simulink model "my_gm_HDLHeaderFull"  (R2024a)
settings: Solver=FixedStepDiscrete  StartTime=0.0  StopTime=stopTime  RelTol=1e-3
values from neighbouring files (symbols this model uses):
  fs = 1    [testHeaderFull.m]
undefined symbols (not defined in the file or in its folder): fPHY, headerBitsPerOFDMSymbol, paramFile
libraries: hdlmdlgenlib x56, simulink x7, dspsrcs4 x5, whdlutilities x5, hdlsllib x3, dspsigops x3, commhdlcrc x1, whdledac x1, HDL_ieee_8021513 x1
settings Model: Creator=cotti  LastModifiedBy=cotti
settings OptimizationCC: BlockReduction=off  ConditionallyExecuteInputs=off  DefaultParameterBehavior=Inlined  InheritOutputTypeSmallerThanSingle=on
settings DebuggingCC: AlgebraicLoopMsg=error  ArtificialAlgebraicLoopMsg=error  InheritedTsInSrcMsg=none  SingleTaskRateTransMsg=error  UnconnectedInputMsg=warning  UnconnectedOutputMsg=warning  UnconnectedLineMsg=warning
settings HardwareCC: ProdBitPerPointer=32  ProdBitPerSizeT=32  ProdBitPerPtrDiffT=32  ProdLargestAtomicFloat=None  ProdIntDivRoundTo=Undefined  ProdEndianess=Unspecified  ProdWordSize=32  ProdHWDeviceType=ASIC/FPGA->ASIC/FPGA  TargetBitPerLong=64  TargetBitPerPointer=64  TargetBitPerSizeT=64  TargetBitPerPtrDiffT=64  TargetLongLongMode=on  TargetIntDivRoundTo=Zero  TargetEndianess=LittleEndian  TargetWordSize=64  TargetHWDeviceType=Custom Processor->MATLAB Host Computer  ProdEqTarget=off

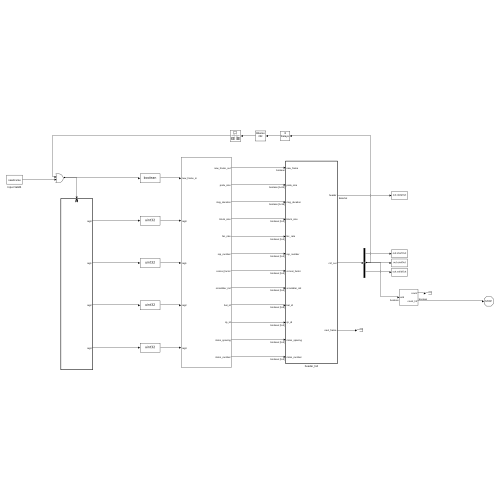
[thumbnail: Simulink's stored preview of the top-level diagram]
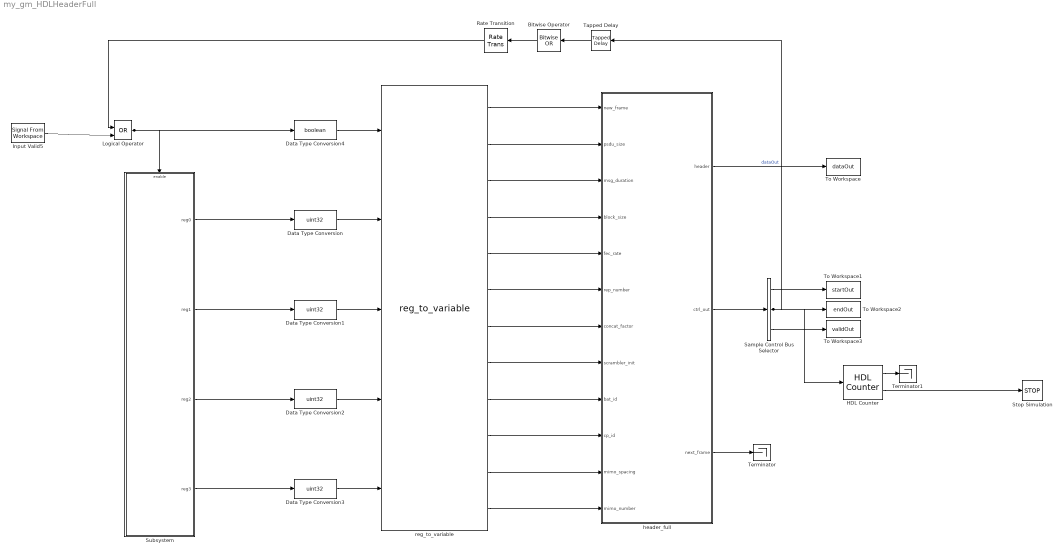
== system my_gm_HDLHeaderFull ==
  Bitwise Operator : simulink/Logic and Bit Operations/Bitwise Operator  logicop=OR  UseBitMask=off  BitMask=bin2dec('11011001')  BitMaskRealWorld=Stored Integer
      settings: LibrarySourceBlock=|
      | hdlsllib/Logic and Bit
      | Operations/Bitwise
      | Operator
  Data Type Conversion{,1..3} (4 alike) : DataTypeConversion  OutDataTypeStr=uint32  SaturateOnIntegerOverflow=off  RndMeth=Floor
  Data Type Conversion4 : DataTypeConversion  OutDataTypeStr=boolean  SaturateOnIntegerOverflow=off  RndMeth=Floor
  HDL Counter : hdlsllib/Sources/HDL Counter  CountType=Count limited  CountInit=0  CountStep=1  CountMax=length(paramFile)  CountFromType=Initial value  CountFrom=0  CountResetPort=off  CountLoadPort=off  CountEnbPort=on  CountDirPort=off  CountHitOutputPort=on  CountDataType=Unsigned  CountWordLen=8  CountFracLen=0  CountSampTime=1
  Input Valid5 : dspsrcs4/Signal From Workspace  X=newFrame  Ts=1/(fPHY/4)  nsamps=1  OutputAfterFinalValue=Setting to zero  ignoreOrWarnInputAndFrameLengths=off  OutputFrames=off
  Logical Operator : Logic  Operator=OR  IconShape=distinctive  AllPortsSameDT=off  OutDataTypeStr=boolean
  Rate Transition : RateTransition  OutPortSampleTimeOpt=Multiple of input port sample time  OutPortSampleTimeMultiple=8
  Sample Control Bus Selector : whdlutilities/Sample Control Bus Selector  OutputSignals=start,end,valid
  Stop Simulation : Stop
  Subsystem : Subsystem
  Tapped Delay : simulink/Discrete/Tapped Delay  vinit=0.0  samptime=-1  NumDelays=8  DelayOrder=Oldest  includeCurrent=off
      settings: LibrarySourceBlock=hdlsllib/Discrete/Tapped Delay
  Terminator : Terminator
  Terminator1 : Terminator
  To Workspace : ToWorkspace  VariableName=dataOut  SampleTime=1/fs
      settings: Save2DSignal=2-D array (concatenate along first dimension)
  To Workspace1 : ToWorkspace  VariableName=startOut  SampleTime=1/fs
      settings: Save2DSignal=2-D array (concatenate along first dimension)
  To Workspace2 : ToWorkspace  VariableName=endOut  SampleTime=1/fs
      settings: Save2DSignal=2-D array (concatenate along first dimension)
  To Workspace3 : ToWorkspace  VariableName=validOut  SampleTime=1/fs
      settings: Save2DSignal=2-D array (concatenate along first dimension)
  header_full : Subsystem  TreatAsAtomicUnit=on
  reg_to_variable : HDL_ieee_8021513/reg_to_variable  SystemSampleTime=-1  VariantActivationTime=update diagram  AllowFlexibleInterface=on  Latency=0  AutoFrameSizeCalculation=off
      settings: SourceProductName=HDL IEEE 8021513
  wires:
  HDL Counter/2 -> Stop Simulation/1
  HDL Counter/1 -> Terminator1/1
  Subsystem/4(reg3) -> Data Type Conversion3/1
  Subsystem/3(reg2) -> Data Type Conversion2/1
  Subsystem/2(reg1) -> Data Type Conversion1/1
  Subsystem/1(reg0) -> Data Type Conversion/1
  Rate Transition/1 -> Logical Operator/1
  Bitwise Operator/1 -> Rate Transition/1
  Tapped Delay/1 -> Bitwise Operator/1
  Input Valid5/1 -> Logical Operator/2
  Logical Operator/1 -> Data Type Conversion4/1, Subsystem/Enable
  header_full/3(next_frame) -> Terminator/1
  Data Type Conversion4/1 -> reg_to_variable/1
  Data Type Conversion3/1 -> reg_to_variable/5
  Data Type Conversion2/1 -> reg_to_variable/4
  Data Type Conversion1/1 -> reg_to_variable/3
  Data Type Conversion/1 -> reg_to_variable/2
  header_full/2(ctrl_out) -> Sample Control Bus Selector/1
  Sample Control Bus Selector/1 -> To Workspace1/1
  Sample Control Bus Selector/3 -> To Workspace3/1
  header_full/1(header) -> To Workspace/1  "dataOut"
  Sample Control Bus Selector/2 -> To Workspace2/1, Tapped Delay/1, HDL Counter/1
  reg_to_variable/1 -> header_full/1(new_frame)
  reg_to_variable/3 -> header_full/3(msg_duration)
  reg_to_variable/4 -> header_full/4(block_size)
  reg_to_variable/5 -> header_full/5(fec_rate)
  reg_to_variable/6 -> header_full/6(rep_number)
  reg_to_variable/7 -> header_full/7(concat_factor)
  reg_to_variable/8 -> header_full/8(scrambler_init)
  reg_to_variable/9 -> header_full/9(bat_id)
  reg_to_variable/10 -> header_full/10(cp_id)
  reg_to_variable/11 -> header_full/11(mimo_spacing)
  reg_to_variable/2 -> header_full/2(psdu_size)
  reg_to_variable/12 -> header_full/12(mimo_number)

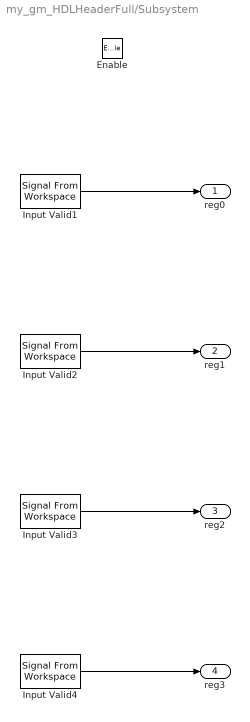
== system my_gm_HDLHeaderFull/Subsystem ==
  Enable : EnablePort
  Input Valid1 : dspsrcs4/Signal From Workspace  X=reg0  Ts=1/(fPHY/4)  nsamps=1  OutputAfterFinalValue=Setting to zero  ignoreOrWarnInputAndFrameLengths=off  OutputFrames=off
  Input Valid2 : dspsrcs4/Signal From Workspace  X=reg1  Ts=1/(fPHY/4)  nsamps=1  OutputAfterFinalValue=Setting to zero  ignoreOrWarnInputAndFrameLengths=off  OutputFrames=off
  Input Valid3 : dspsrcs4/Signal From Workspace  X=reg2  Ts=1/(fPHY/4)  nsamps=1  OutputAfterFinalValue=Setting to zero  ignoreOrWarnInputAndFrameLengths=off  OutputFrames=off
  Input Valid4 : dspsrcs4/Signal From Workspace  X=reg3  Ts=1/(fPHY/4)  nsamps=1  OutputAfterFinalValue=Setting to zero  ignoreOrWarnInputAndFrameLengths=off  OutputFrames=off
  reg0 : Outport
  reg1 : Outport  Port=2
  reg2 : Outport  Port=3
  reg3 : Outport  Port=4
  wires:
  Input Valid1/1 -> reg0/1
  Input Valid4/1 -> reg3/1
  Input Valid2/1 -> reg1/1
  Input Valid3/1 -> reg2/1

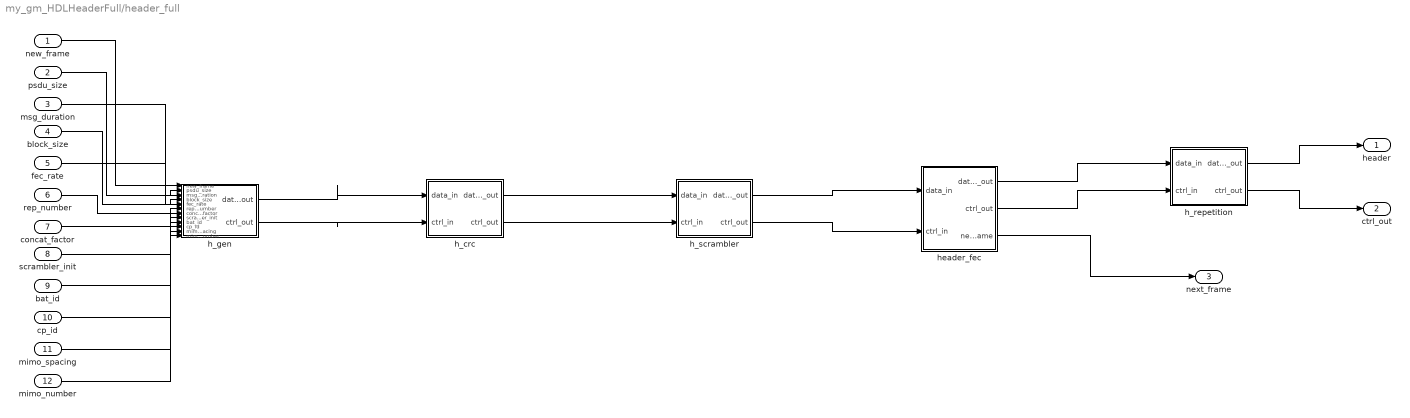
== system my_gm_HDLHeaderFull/header_full ==
  new_frame : Inport  OutDataTypeStr=boolean  SampleTime=8e-08
  psdu_size : Inport  Port=2  OutDataTypeStr=boolean  PortDimensions=[1 24]  SampleTime=8e-08
  msg_duration : Inport  Port=3  OutDataTypeStr=boolean  PortDimensions=[1 16]  SampleTime=8e-08
  block_size : Inport  Port=4  OutDataTypeStr=boolean  PortDimensions=[1 2]  SampleTime=8e-08
  fec_rate : Inport  Port=5  OutDataTypeStr=boolean  PortDimensions=[1 3]  SampleTime=8e-08
  rep_number : Inport  Port=6  OutDataTypeStr=boolean  PortDimensions=[1 3]  SampleTime=8e-08
  concat_factor : Inport  Port=7  OutDataTypeStr=boolean  PortDimensions=[1 3]  SampleTime=8e-08
  scrambler_init : Inport  Port=8  OutDataTypeStr=boolean  PortDimensions=[1 4]  SampleTime=8e-08
  bat_id : Inport  Port=9  OutDataTypeStr=boolean  PortDimensions=[1 5]  SampleTime=8e-08
  cp_id : Inport  Port=10  OutDataTypeStr=boolean  PortDimensions=[1 3]  SampleTime=8e-08
  mimo_spacing : Inport  Port=11  OutDataTypeStr=boolean  PortDimensions=[1 3]  SampleTime=8e-08
  mimo_number : Inport  Port=12  OutDataTypeStr=boolean  PortDimensions=[1 3]  SampleTime=8e-08
  h_crc : Subsystem
  h_gen : Subsystem
  h_repetition : Subsystem
  h_scrambler : Subsystem
  header_fec : Subsystem
  header : Outport  SampleTime=1e-08
  ctrl_out : Outport  Port=2  SampleTime=1e-08
  next_frame : Outport  Port=3  SampleTime=1e-08
  wires:
  new_frame/1 -> h_gen/1(new_frame)
  psdu_size/1 -> h_gen/2(psdu_size)
  msg_duration/1 -> h_gen/3(msg_duration)
  block_size/1 -> h_gen/4(block_size)
  fec_rate/1 -> h_gen/5(fec_rate)
  rep_number/1 -> h_gen/6(rep_number)
  concat_factor/1 -> h_gen/7(concat_factor)
  scrambler_init/1 -> h_gen/8(scrambler_init)
  bat_id/1 -> h_gen/9(bat_id)
  cp_id/1 -> h_gen/10(cp_id)
  mimo_spacing/1 -> h_gen/11(mimo_spacing)
  mimo_number/1 -> h_gen/12(mimo_number)
  h_crc/1(data_out) -> h_scrambler/1(data_in)
  h_crc/2(ctrl_out) -> h_scrambler/2(ctrl_in)
  h_gen/1(data_out) -> h_crc/1(data_in)
  h_gen/2(ctrl_out) -> h_crc/2(ctrl_in)
  h_repetition/1(data_out) -> header/1
  h_repetition/2(ctrl_out) -> ctrl_out/1
  h_scrambler/1(data_out) -> header_fec/1(data_in)
  h_scrambler/2(ctrl_out) -> header_fec/2(ctrl_in)
  header_fec/1(data_out) -> h_repetition/1(data_in)
  header_fec/2(ctrl_out) -> h_repetition/2(ctrl_in)
  header_fec/3(next_frame) -> next_frame/1

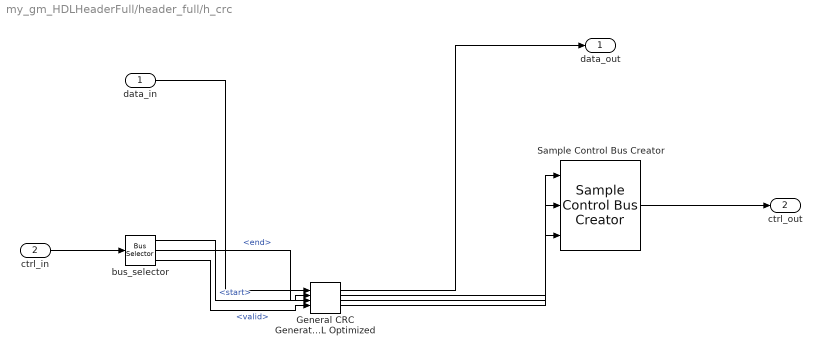
== system my_gm_HDLHeaderFull/header_full/h_crc ==
  data_in : Inport  OutDataTypeStr=boolean  SampleTime=1e-08
  ctrl_in : Inport  Port=2  SampleTime=1e-08
  General CRC Generator HDL Optimized : commhdlcrc/General CRC Generator HDL Optimized  Polynomial=headerCRCPoly  InitialState=1  DirectMethod=on  ReflectInput=off  ReflectCRCChecksum=off  FinalXORValue=0  SimulateUsing=Code generation
  Sample Control Bus Creator : whdlutilities/Sample Control Bus Creator
  bus_selector : BusSelector  OutputSignals=start,end,valid
  data_out : Outport  SampleTime=1e-08
  ctrl_out : Outport  Port=2  SampleTime=1e-08
  wires:
  data_in/1 -> General CRC Generator HDL Optimized/1
  ctrl_in/1 -> bus_selector/1
  General CRC Generator HDL Optimized/1 -> data_out/1
  General CRC Generator HDL Optimized/2 -> Sample Control Bus Creator/1
  General CRC Generator HDL Optimized/3 -> Sample Control Bus Creator/2
  General CRC Generator HDL Optimized/4 -> Sample Control Bus Creator/3
  Sample Control Bus Creator/1 -> ctrl_out/1
  bus_selector/1 -> General CRC Generator HDL Optimized/2  "<start>"
  bus_selector/2 -> General CRC Generator HDL Optimized/3  "<end>"
  bus_selector/3 -> General CRC Generator HDL Optimized/4  "<valid>"

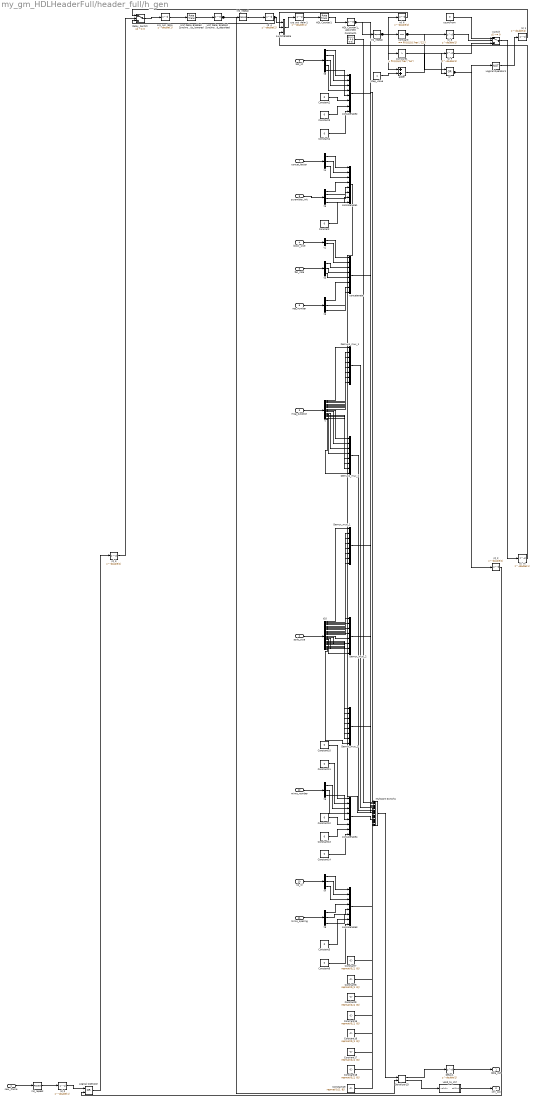
== system my_gm_HDLHeaderFull/header_full/h_gen ==
  new_frame : Inport  OutDataTypeStr=boolean  SampleTime=8e-08
  psdu_size : Inport  Port=2  OutDataTypeStr=boolean  PortDimensions=[1 24]  SampleTime=8e-08
  msg_duration : Inport  Port=3  OutDataTypeStr=boolean  PortDimensions=[1 16]  SampleTime=8e-08
  block_size : Inport  Port=4  OutDataTypeStr=boolean  PortDimensions=[1 2]  SampleTime=8e-08
  fec_rate : Inport  Port=5  OutDataTypeStr=boolean  PortDimensions=[1 3]  SampleTime=8e-08
  rep_number : Inport  Port=6  OutDataTypeStr=boolean  PortDimensions=[1 3]  SampleTime=8e-08
  concat_factor : Inport  Port=7  OutDataTypeStr=boolean  PortDimensions=[1 3]  SampleTime=8e-08
  scrambler_init : Inport  Port=8  OutDataTypeStr=boolean  PortDimensions=[1 4]  SampleTime=8e-08
  bat_id : Inport  Port=9  OutDataTypeStr=boolean  PortDimensions=[1 5]  SampleTime=8e-08
  cp_id : Inport  Port=10  OutDataTypeStr=boolean  PortDimensions=[1 3]  SampleTime=8e-08
  mimo_spacing : Inport  Port=11  OutDataTypeStr=boolean  PortDimensions=[1 3]  SampleTime=8e-08
  mimo_number : Inport  Port=12  OutDataTypeStr=boolean  PortDimensions=[1 3]  SampleTime=8e-08
  Constant{,2..6,10..14} (11 alike) : Constant  Value=0  OutDataTypeStr=boolean  SampleTime=8e-08
  Constant1 : Constant  Value=[0 0 1 1 0 0 0 0]  VectorParams1D=off  OutDataTypeStr=boolean  SampleTime=8e-08
  Constant{7..9,15..19} (8 alike) : Constant  Value="repmat(0,[1  8])"  VectorParams1D=off  OutDataTypeStr=boolean  SampleTime=8e-08
  Delay1 : Delay  DelayLength=double(1)  InitialCondition=0  SampleTime=1e-08
  Delay_Switch : Switch  Criteria=u2 ~= 0  Threshold=double(0)  OutDataTypeStr=boolean  SampleTime=1e-08  SaturateOnIntegerOverflow=off  InputSameDT=off
  Demux1_mux_1 : Mux  Inputs=8
  Demux1_mux_2 : Mux  Inputs=8
  Demux_mux_1 : Mux  Inputs=8
  Demux_mux_2 : Mux  Inputs=8
  Demux_mux_3 : Mux  Inputs=8
  HDL Counter1 : RateTransition  OutPortSampleTimeOpt=Multiple of input port sample time  OutPortSampleTimeMultiple=8
  HDL Counter1_absorbed : Delay  DelayLength=0
  Logical Operator : Logic  Operator=OR  AllPortsSameDT=off  OutDataTypeStr=boolean  SampleTime=1e-08
  Logical Operator1 : Logic  Operator=NOT  Inputs=1  AllPortsSameDT=off  OutDataTypeStr=boolean  SampleTime=1e-08
  Multiport Switch1 : MultiPortSwitch  DataPortOrder=Zero-based contiguous  Inputs=19  DiagnosticForDefault=None  zeroidx=on  SampleTime=8e-08  SaturateOnIntegerOverflow=off  InputSameDT=off
  Serializer1D : hdlsllib/HDL Operations/Serializer1D  Ratio=8  IdleCycles=0  validIn=on  startOut=off  validOut=on  inputDataDimensions=8  inputSampleTime=8e-08  inputSignalType=real
  Unit Delay Enabled Synchronous_lowered : RateTransition  OutPortSampleTimeOpt=Multiple of input port sample time  OutPortSampleTimeMultiple=8
  Unit Delay Enabled Synchronous_lowered_absorbed : Delay  DelayLength=0
  adder : Sum  OutDataTypeStr=fixdt(0, 5, 0)  AccumDataTypeStr=fixdt(0, 5, 0)  SampleTime=1e-08
  compare : simulink/Logic and Bit Operations/Compare To Constant  relop===  const="fi(0,0,5,0,\"hex\",\"12\")"  OutDataTypeStr=boolean
  compare1 : simulink/Logic and Bit Operations/Compare To Constant  relop=>  const="fi(0,0,5,0,\"hex\",\"1e\")"  OutDataTypeStr=boolean
  concatenate{,1..4} (5 alike) : Concatenate  NumInputs=8  Mode=Multidimensional array  ConcatenateDimension=2
  countFrom : Constant  Value=0  VectorParams1D=off  OutDataTypeStr=fixdt(0, 5, 0)  SampleTime=1e-08
  crp_out_delay : Delay  DelayLength=double(1)  InitialCondition=0  SampleTime=1e-08
  crp_out_delay1 : Delay  DelayLength=double(1)  InitialCondition=0  SampleTime=1e-08
  in0_repeat : dspsigops/Repeat  FactorSource=Dialog parameter  N=double(8)  Nmax=16  RateOptions=Allow multirate processing  ic=0  mode=Unused parameter value
  in1_repeat : dspsigops/Repeat  FactorSource=Dialog parameter  N=double(8)  Nmax=16  RateOptions=Allow multirate processing  ic=0  mode=Unused parameter value
  in2_repeat : dspsigops/Repeat  FactorSource=Dialog parameter  N=double(8)  Nmax=16  RateOptions=Allow multirate processing  ic=0  mode=Unused parameter value
  or : Logic  Operator=OR  AllPortsSameDT=off  OutDataTypeStr=boolean  SampleTime=1e-08
  rd_{0,2..3,8..10} (6 alike) : Delay  DelayLength=double(1)  InitialCondition=0  SampleTime=1e-08
  rd_1 : Delay  DelayLength=double(2)  InitialCondition=0  SampleTime=1e-08
  rd_4 : Delay  DelayLength=double(2)  InitialCondition=0  SampleTime=1e-08
  rd_6 : Delay  DelayLength=double(2)  InitialCondition=0  SampleTime=1e-08
  step_value : Constant  VectorParams1D=off  OutDataTypeStr=fixdt(0, 5, 0)  SampleTime=1e-08
  switch : Switch  Criteria=u2 ~= 0  Threshold=double(0)  OutDataTypeStr=fixdt(0, 5, 0)  SampleTime=1e-08  SaturateOnIntegerOverflow=off  InputSameDT=off
  switchEnable : MultiPortSwitch  DataPortOrder=Zero-based contiguous  Inputs=2  DiagnosticForDefault=None  zeroidx=on  OutDataTypeStr=fixdt(0, 5, 0)  SampleTime=1e-08  SaturateOnIntegerOverflow=off  InputSameDT=off
  t : Demux  Outputs=16
  t1 : Demux  Outputs=2
  t10 : Demux  Outputs=24
  t{2..4,7..9} (6 alike) : Demux  Outputs=3
  t5 : Demux
  t6 : Demux  Outputs=5
  valid_to_ctrl : Subsystem
  data_out : Outport  SampleTime=1e-08
  ctrl_out : Outport  Port=2  SampleTime=1e-08
  wires:
  new_frame/1 -> in2_repeat/1
  psdu_size/1 -> t10/1
  msg_duration/1 -> t/1
  block_size/1 -> t1/1
  fec_rate/1 -> t2/1
  rep_number/1 -> t3/1
  concat_factor/1 -> t4/1
  scrambler_init/1 -> t5/1
  bat_id/1 -> t6/1
  cp_id/1 -> t7/1
  mimo_spacing/1 -> t8/1
  mimo_number/1 -> t9/1
  Delay1/1 -> data_out/1
  valid_to_ctrl/1(ctrlOut) -> ctrl_out/1
  Serializer1D/2 -> valid_to_ctrl/1(validIn)
  Serializer1D/1 -> Delay1/1
  Constant1/1 -> Multiport Switch1/2
  Demux1_mux_1/1 -> Multiport Switch1/6
  Demux1_mux_2/1 -> Multiport Switch1/7
  concatenate/1 -> Multiport Switch1/8
  Constant/1 -> concatenate1/8
  concatenate1/1 -> Multiport Switch1/9
  Constant2/1 -> concatenate2/6
  Constant3/1 -> concatenate2/7
  Constant4/1 -> concatenate2/8
  concatenate2/1 -> Multiport Switch1/10
  Constant5/1 -> concatenate3/7
  Constant6/1 -> concatenate3/8
  concatenate3/1 -> Multiport Switch1/11
  Constant7/1 -> Multiport Switch1/12
  Constant8/1 -> Multiport Switch1/13
  Constant9/1 -> Multiport Switch1/14
  Constant10/1 -> concatenate4/1
  Constant11/1 -> concatenate4/2
  Constant12/1 -> concatenate4/6
  Constant13/1 -> concatenate4/7
  Constant14/1 -> concatenate4/8
  concatenate4/1 -> Multiport Switch1/15
  Constant15/1 -> Multiport Switch1/16
  Constant16/1 -> Multiport Switch1/17
  Constant17/1 -> Multiport Switch1/18
  Constant18/1 -> Multiport Switch1/19
  Constant19/1 -> Multiport Switch1/20
  Multiport Switch1/1 -> Serializer1D/1
  Demux_mux_1/1 -> Multiport Switch1/3
  Demux_mux_2/1 -> Multiport Switch1/4
  Demux_mux_3/1 -> Multiport Switch1/5
  t/1 -> Demux1_mux_1/1
  t/2 -> Demux1_mux_1/2
  t/3 -> Demux1_mux_1/3
  t/4 -> Demux1_mux_1/4
  t/5 -> Demux1_mux_1/5
  t/6 -> Demux1_mux_1/6
  t/7 -> Demux1_mux_1/7
  t/8 -> Demux1_mux_1/8
  t/9 -> Demux1_mux_2/1
  t/10 -> Demux1_mux_2/2
  t/11 -> Demux1_mux_2/3
  t/12 -> Demux1_mux_2/4
  t/13 -> Demux1_mux_2/5
  t/14 -> Demux1_mux_2/6
  t/15 -> Demux1_mux_2/7
  t/16 -> Demux1_mux_2/8
  t1/1 -> concatenate/1
  t1/2 -> concatenate/2
  t2/1 -> concatenate/3
  t2/2 -> concatenate/4
  t2/3 -> concatenate/5
  t3/1 -> concatenate/6
  t3/2 -> concatenate/7
  t3/3 -> concatenate/8
  t4/1 -> concatenate1/1
  t4/2 -> concatenate1/2
  t4/3 -> concatenate1/3
  t5/1 -> concatenate1/4
  t5/2 -> concatenate1/5
  t5/3 -> concatenate1/6
  t5/4 -> concatenate1/7
  t6/1 -> concatenate2/1
  t6/2 -> concatenate2/2
  t6/3 -> concatenate2/3
  t6/4 -> concatenate2/4
  t6/5 -> concatenate2/5
  t7/1 -> concatenate3/1
  t7/2 -> concatenate3/2
  t7/3 -> concatenate3/3
  t8/1 -> concatenate3/4
  t8/2 -> concatenate3/5
  t8/3 -> concatenate3/6
  t9/1 -> concatenate4/3
  t9/2 -> concatenate4/4
  t9/3 -> concatenate4/5
  t10/1 -> Demux_mux_1/1
  t10/2 -> Demux_mux_1/2
  t10/3 -> Demux_mux_1/3
  t10/4 -> Demux_mux_1/4
  t10/5 -> Demux_mux_1/5
  t10/6 -> Demux_mux_1/6
  t10/7 -> Demux_mux_1/7
  t10/8 -> Demux_mux_1/8
  t10/9 -> Demux_mux_2/1
  t10/10 -> Demux_mux_2/2
  t10/11 -> Demux_mux_2/3
  t10/12 -> Demux_mux_2/4
  t10/13 -> Demux_mux_2/5
  t10/14 -> Demux_mux_2/6
  t10/15 -> Demux_mux_2/7
  t10/16 -> Demux_mux_2/8
  t10/17 -> Demux_mux_3/1
  t10/18 -> Demux_mux_3/2
  t10/19 -> Demux_mux_3/3
  t10/20 -> Demux_mux_3/4
  t10/21 -> Demux_mux_3/5
  t10/22 -> Demux_mux_3/6
  t10/23 -> Demux_mux_3/7
  t10/24 -> Demux_mux_3/8
  Unit Delay Enabled Synchronous_lowered_absorbed/1 -> Serializer1D/2, in0_repeat/1
  in2_repeat/1 -> rd_0/1
  HDL Counter1/1 -> HDL Counter1_absorbed/1
  HDL Counter1_absorbed/1 -> Multiport Switch1/1, in1_repeat/1
  in1_repeat/1 -> rd_6/1, adder/1, compare/1, compare1/1
  in0_repeat/1 -> rd_4/1
  crp_out_delay/1 -> Unit Delay Enabled Synchronous_lowered/1
  crp_out_delay1/1 -> HDL Counter1/1
  Unit Delay Enabled Synchronous_lowered/1 -> Unit Delay Enabled Synchronous_lowered_absorbed/1
  switchEnable/1 -> crp_out_delay1/1
  countFrom/1 -> switch/1
  step_value/1 -> adder/2
  adder/1 -> rd_9/1
  switch/1 -> rd_10/1
  compare/1 -> rd_8/1, or/1
  compare1/1 -> or/2
  or/1 -> rd_2/1, Logical Operator1/1
  Logical Operator1/1 -> rd_1/1
  Delay_Switch/1 -> crp_out_delay/1
  Logical Operator/1 -> rd_3/1
  rd_6/1 -> switchEnable/2
  rd_1/1 -> Delay_Switch/1
  rd_0/1 -> Logical Operator/1
  rd_2/1 -> Logical Operator/2
  rd_3/1 -> Delay_Switch/2
  rd_9/1 -> switch/3
  rd_10/1 -> switchEnable/3
  rd_8/1 -> switch/2
  rd_4/1 -> Delay_Switch/3, switchEnable/1

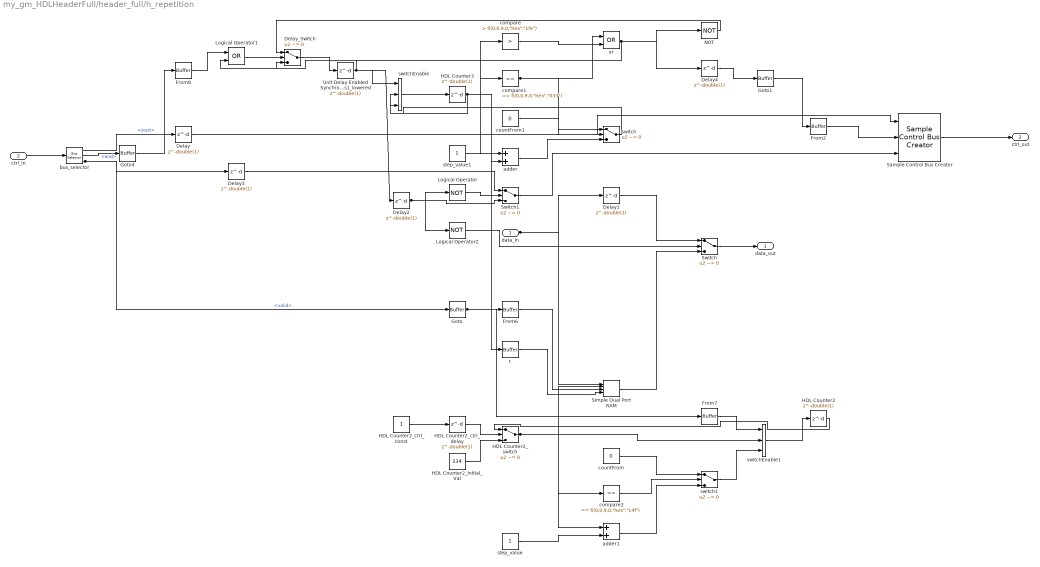
== system my_gm_HDLHeaderFull/header_full/h_repetition ==
  data_in : Inport  OutDataTypeStr=boolean  SampleTime=1e-08
  ctrl_in : Inport  Port=2  SampleTime=1e-08
  Delay{,1..4} (5 alike) : Delay  DelayLength=double(1)  InitialCondition=0  SampleTime=1e-08
  Delay_Switch : Switch  Criteria=u2 ~= 0  Threshold=double(0)  OutDataTypeStr=boolean  SampleTime=1e-08  SaturateOnIntegerOverflow=off  InputSameDT=off
  From{2,6..8} (4 alike) : hdlmdlgenlib/Buffer
  Goto : hdlmdlgenlib/Buffer
  Goto1 : hdlmdlgenlib/Buffer
  Goto4 : hdlmdlgenlib/Buffer
  HDL Counter2 : Delay  DelayLength=double(1)  InitialCondition=0  SampleTime=1e-08
  HDL Counter2_Initial_Val : Constant  Value=334  OutDataTypeStr=fixdt(0, 9, 0)  SampleTime=1e-08
  HDL Counter2_ctrl_const : Constant  OutDataTypeStr=boolean  SampleTime=1e-08
  HDL Counter2_ctrl_delay : Delay  DelayLength=double(1)  InitialCondition=0  SampleTime=1e-08
  HDL Counter2_switch : Switch  Criteria=u2 ~= 0  Threshold=double(0)  OutDataTypeStr=fixdt(0, 9, 0)  SampleTime=1e-08  SaturateOnIntegerOverflow=off  InputSameDT=off
  HDL Counter3 : Delay  DelayLength=double(1)  InitialCondition=0  SampleTime=1e-08
  Logical Operator : Logic  Operator=NOT  Inputs=1  AllPortsSameDT=off  OutDataTypeStr=boolean  SampleTime=1e-08
  Logical Operator1 : Logic  Operator=OR  AllPortsSameDT=off  OutDataTypeStr=boolean  SampleTime=1e-08
  Logical Operator2 : Logic  Operator=NOT  Inputs=1  AllPortsSameDT=off  OutDataTypeStr=boolean  SampleTime=1e-08
  NOT : Logic  Operator=NOT  Inputs=1  AllPortsSameDT=off  OutDataTypeStr=boolean  SampleTime=1e-08
  Sample Control Bus Creator : whdlutilities/Sample Control Bus Creator
  Simple Dual Port RAM : hdlsllib/HDL RAMs/Simple Dual Port RAM  ram_size=nextpow2(headerBitsPerOFDMSymbol)
  Switch : Switch  Criteria=u2 ~= 0  Threshold=double(0)  OutDataTypeStr=boolean  SampleTime=1e-08  SaturateOnIntegerOverflow=off  InputSameDT=off
  Switch1 : Switch  Criteria=u2 ~= 0  Threshold=double(0)  OutDataTypeStr=boolean  SampleTime=1e-08  SaturateOnIntegerOverflow=off  InputSameDT=off
  Unit Delay Enabled Synchronous1_lowered : Delay  DelayLength=double(1)  InitialCondition=0  SampleTime=1e-08
  adder : Sum  OutDataTypeStr=fixdt(0, 9, 0)  AccumDataTypeStr=fixdt(0, 9, 0)  SampleTime=1e-08
  adder1 : Sum  OutDataTypeStr=fixdt(0, 9, 0)  AccumDataTypeStr=fixdt(0, 9, 0)  SampleTime=1e-08
  bus_selector : BusSelector  OutputSignals=start,end,valid
  compare : simulink/Logic and Bit Operations/Compare To Constant  relop=>  const="fi(0,0,9,0,\"hex\",\"1fe\")"  OutDataTypeStr=boolean
  compare1 : simulink/Logic and Bit Operations/Compare To Constant  relop===  const="fi(0,0,9,0,\"hex\",\"033\")"  OutDataTypeStr=boolean
  compare2 : simulink/Logic and Bit Operations/Compare To Constant  relop===  const="fi(0,0,9,0,\"hex\",\"14f\")"  OutDataTypeStr=boolean
  countFrom : Constant  Value=0  VectorParams1D=off  OutDataTypeStr=fixdt(0, 9, 0)  SampleTime=1e-08
  countFrom1 : Constant  Value=0  VectorParams1D=off  OutDataTypeStr=fixdt(0, 9, 0)  SampleTime=1e-08
  or : Logic  Operator=OR  AllPortsSameDT=off  OutDataTypeStr=boolean  SampleTime=1e-08
  step_value : Constant  VectorParams1D=off  OutDataTypeStr=fixdt(0, 9, 0)  SampleTime=1e-08
  step_value1 : Constant  VectorParams1D=off  OutDataTypeStr=fixdt(0, 9, 0)  SampleTime=1e-08
  switch : Switch  Criteria=u2 ~= 0  Threshold=double(0)  OutDataTypeStr=fixdt(0, 9, 0)  SampleTime=1e-08  SaturateOnIntegerOverflow=off  InputSameDT=off
  switch1 : Switch  Criteria=u2 ~= 0  Threshold=double(0)  OutDataTypeStr=fixdt(0, 9, 0)  SampleTime=1e-08  SaturateOnIntegerOverflow=off  InputSameDT=off
  switchEnable : MultiPortSwitch  DataPortOrder=Zero-based contiguous  Inputs=2  DiagnosticForDefault=None  zeroidx=on  OutDataTypeStr=fixdt(0, 9, 0)  SampleTime=1e-08  SaturateOnIntegerOverflow=off  InputSameDT=off
  switchEnable1 : MultiPortSwitch  DataPortOrder=Zero-based contiguous  Inputs=2  DiagnosticForDefault=None  zeroidx=on  OutDataTypeStr=fixdt(0, 9, 0)  SampleTime=1e-08  SaturateOnIntegerOverflow=off  InputSameDT=off
  t : hdlmdlgenlib/Buffer
  data_out : Outport  SampleTime=1e-08
  ctrl_out : Outport  Port=2  SampleTime=1e-08
  wires:
  data_in/1 -> Delay1/1, Simple Dual Port RAM/1
  ctrl_in/1 -> bus_selector/1
  bus_selector/1 -> Delay/1  "<start>"
  bus_selector/2 -> Goto4/1  "<end>"
  bus_selector/3 -> Goto/1, Delay3/1  "<valid>"
  Delay/1 -> Sample Control Bus Creator/1
  Delay1/1 -> Switch/1
  Delay2/1 -> Switch1/3, Logical Operator2/1, Logical Operator/1
  Delay3/1 -> Switch1/1
  Delay4/1 -> Goto1/1
  From2/1 -> Sample Control Bus Creator/2
  From6/1 -> Simple Dual Port RAM/3
  From7/1 -> switchEnable1/1
  t/1 -> Simple Dual Port RAM/4
  Logical Operator/1 -> Switch1/2
  Logical Operator2/1 -> Switch/2
  Sample Control Bus Creator/1 -> ctrl_out/1
  Simple Dual Port RAM/1 -> Switch/3
  Switch/1 -> data_out/1
  Switch1/1 -> Sample Control Bus Creator/3
  Unit Delay Enabled Synchronous1_lowered/1 -> Delay2/1, switchEnable/1, Delay_Switch/3
  Goto1/1 -> From2/1
  Goto/1 -> From7/1, From6/1
  Goto4/1 -> From8/1
  HDL Counter2_switch/1 -> adder1/1, compare2/1, switchEnable1/2, Simple Dual Port RAM/2
  HDL Counter3/1 -> t/1, adder/1, compare1/1, compare/1, switchEnable/2
  or/1 -> Delay4/1, Logical Operator1/2, NOT/1
  HDL Counter2_ctrl_const/1 -> HDL Counter2_ctrl_delay/1
  step_value1/1 -> adder/2
  countFrom1/1 -> switch/1
  From8/1 -> Logical Operator1/1
  Delay_Switch/1 -> Unit Delay Enabled Synchronous1_lowered/1
  switchEnable/1 -> HDL Counter3/1
  adder/1 -> switch/3
  switch/1 -> switchEnable/3
  Logical Operator1/1 -> Delay_Switch/2
  compare/1 -> or/2
  compare1/1 -> or/1, switch/2
  NOT/1 -> Delay_Switch/1
  HDL Counter2/1 -> HDL Counter2_switch/1
  step_value/1 -> adder1/2
  countFrom/1 -> switch1/1
  HDL Counter2_ctrl_delay/1 -> HDL Counter2_switch/2
  HDL Counter2_Initial_Val/1 -> HDL Counter2_switch/3
  switchEnable1/1 -> HDL Counter2/1
  adder1/1 -> switch1/3
  compare2/1 -> switch1/2
  switch1/1 -> switchEnable1/3

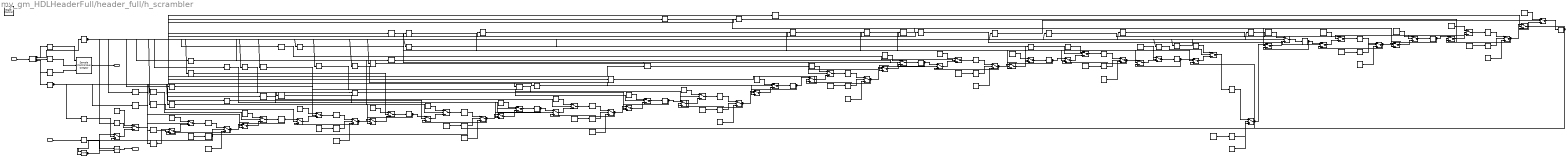
== system my_gm_HDLHeaderFull/header_full/h_scrambler ==
  data_in : Inport  OutDataTypeStr=boolean  SampleTime=1e-08
  ctrl_in : Inport  Port=2  SampleTime=1e-08
  C10_lowered : Delay  DelayLength=double(1)  InitialCondition=0  SampleTime=1e-08
  C10_lowered_Initial_Val : Constant  Value=double(1)  OutDataTypeStr=boolean  SampleTime=1e-08
  C10_lowered_ctrl_const : Constant  OutDataTypeStr=boolean  SampleTime=1e-08
  C10_lowered_ctrl_delay : Delay  DelayLength=double(1)  InitialCondition=0  SampleTime=1e-08
  C10_lowered_switch : Switch  Criteria=u2 ~= 0  Threshold=double(0)  OutDataTypeStr=boolean  SampleTime=1e-08  SaturateOnIntegerOverflow=off  InputSameDT=off
  C11_lowered : Delay  DelayLength=double(1)  InitialCondition=0  SampleTime=1e-08
  C12_lowered : Delay  DelayLength=double(1)  InitialCondition=0  SampleTime=1e-08
  C12_lowered_Initial_Val : Constant  Value=double(1)  OutDataTypeStr=boolean  SampleTime=1e-08
  C12_lowered_ctrl_const : Constant  OutDataTypeStr=boolean  SampleTime=1e-08
  C12_lowered_ctrl_delay : Delay  DelayLength=double(1)  InitialCondition=0  SampleTime=1e-08
  C12_lowered_switch : Switch  Criteria=u2 ~= 0  Threshold=double(0)  OutDataTypeStr=boolean  SampleTime=1e-08  SaturateOnIntegerOverflow=off  InputSameDT=off
  C13_lowered : Delay  DelayLength=double(1)  InitialCondition=0  SampleTime=1e-08
  C14_lowered : Delay  DelayLength=double(1)  InitialCondition=0  SampleTime=1e-08
  C14_lowered_Initial_Val : Constant  Value=double(1)  OutDataTypeStr=boolean  SampleTime=1e-08
  C14_lowered_ctrl_const : Constant  OutDataTypeStr=boolean  SampleTime=1e-08
  C14_lowered_ctrl_delay : Delay  DelayLength=double(1)  InitialCondition=0  SampleTime=1e-08
  C14_lowered_switch : Switch  Criteria=u2 ~= 0  Threshold=double(0)  OutDataTypeStr=boolean  SampleTime=1e-08  SaturateOnIntegerOverflow=off  InputSameDT=off
  C15_lowered : Delay  DelayLength=double(1)  InitialCondition=0  SampleTime=1e-08
  C16_lowered : Delay  DelayLength=double(1)  InitialCondition=0  SampleTime=1e-08
  C16_lowered_Initial_Val : Constant  Value=double(1)  OutDataTypeStr=boolean  SampleTime=1e-08
  C16_lowered_ctrl_const : Constant  OutDataTypeStr=boolean  SampleTime=1e-08
  C16_lowered_ctrl_delay : Delay  DelayLength=double(1)  InitialCondition=0  SampleTime=1e-08
  C16_lowered_switch : Switch  Criteria=u2 ~= 0  Threshold=double(0)  OutDataTypeStr=boolean  SampleTime=1e-08  SaturateOnIntegerOverflow=off  InputSameDT=off
  C17_lowered : Delay  DelayLength=double(1)  InitialCondition=0  SampleTime=1e-08
  C18_lowered : Delay  DelayLength=double(1)  InitialCondition=0  SampleTime=1e-08
  C18_lowered_Initial_Val : Constant  Value=double(1)  OutDataTypeStr=boolean  SampleTime=1e-08
  C18_lowered_ctrl_const : Constant  OutDataTypeStr=boolean  SampleTime=1e-08
  C18_lowered_ctrl_delay : Delay  DelayLength=double(1)  InitialCondition=0  SampleTime=1e-08
  C18_lowered_switch : Switch  Criteria=u2 ~= 0  Threshold=double(0)  OutDataTypeStr=boolean  SampleTime=1e-08  SaturateOnIntegerOverflow=off  InputSameDT=off
  C19_lowered : Delay  DelayLength=double(1)  InitialCondition=0  SampleTime=1e-08
  C1_lowered : Delay  DelayLength=double(1)  InitialCondition=0  SampleTime=1e-08
  C20_lowered : Delay  DelayLength=double(1)  InitialCondition=0  SampleTime=1e-08
  C20_lowered_Initial_Val : Constant  Value=double(1)  OutDataTypeStr=boolean  SampleTime=1e-08
  C20_lowered_ctrl_const : Constant  OutDataTypeStr=boolean  SampleTime=1e-08
  C20_lowered_ctrl_delay : Delay  DelayLength=double(1)  InitialCondition=0  SampleTime=1e-08
  C20_lowered_switch : Switch  Criteria=u2 ~= 0  Threshold=double(0)  OutDataTypeStr=boolean  SampleTime=1e-08  SaturateOnIntegerOverflow=off  InputSameDT=off
  C21_lowered : Delay  DelayLength=double(1)  InitialCondition=0  SampleTime=1e-08
  C22_lowered : Delay  DelayLength=double(1)  InitialCondition=0  SampleTime=1e-08
  C22_lowered_Initial_Val : Constant  Value=double(1)  OutDataTypeStr=boolean  SampleTime=1e-08
  C22_lowered_ctrl_const : Constant  OutDataTypeStr=boolean  SampleTime=1e-08
  C22_lowered_ctrl_delay : Delay  DelayLength=double(1)  InitialCondition=0  SampleTime=1e-08
  C22_lowered_switch : Switch  Criteria=u2 ~= 0  Threshold=double(0)  OutDataTypeStr=boolean  SampleTime=1e-08  SaturateOnIntegerOverflow=off  InputSameDT=off
  C23_lowered : Delay  DelayLength=double(1)  InitialCondition=0  SampleTime=1e-08
  C2_lowered : Delay  DelayLength=double(1)  InitialCondition=0  SampleTime=1e-08
  C2_lowered_Initial_Val : Constant  Value=double(1)  OutDataTypeStr=boolean  SampleTime=1e-08
  C2_lowered_ctrl_const : Constant  OutDataTypeStr=boolean  SampleTime=1e-08
  C2_lowered_ctrl_delay : Delay  DelayLength=double(1)  InitialCondition=0  SampleTime=1e-08
  C2_lowered_switch : Switch  Criteria=u2 ~= 0  Threshold=double(0)  OutDataTypeStr=boolean  SampleTime=1e-08  SaturateOnIntegerOverflow=off  InputSameDT=off
  C3_lowered : Delay  DelayLength=double(1)  InitialCondition=0  SampleTime=1e-08
  C4_lowered : Delay  DelayLength=double(1)  InitialCondition=0  SampleTime=1e-08
  C4_lowered_Initial_Val : Constant  Value=double(1)  OutDataTypeStr=boolean  SampleTime=1e-08
  C4_lowered_ctrl_const : Constant  OutDataTypeStr=boolean  SampleTime=1e-08
  C4_lowered_ctrl_delay : Delay  DelayLength=double(1)  InitialCondition=0  SampleTime=1e-08
  C4_lowered_switch : Switch  Criteria=u2 ~= 0  Threshold=double(0)  OutDataTypeStr=boolean  SampleTime=1e-08  SaturateOnIntegerOverflow=off  InputSameDT=off
  C5_lowered : Delay  DelayLength=double(1)  InitialCondition=0  SampleTime=1e-08
  C6_lowered : Delay  DelayLength=double(1)  InitialCondition=0  SampleTime=1e-08
  C6_lowered_Initial_Val : Constant  Value=double(1)  OutDataTypeStr=boolean  SampleTime=1e-08
  C6_lowered_ctrl_const : Constant  OutDataTypeStr=boolean  SampleTime=1e-08
  C6_lowered_ctrl_delay : Delay  DelayLength=double(1)  InitialCondition=0  SampleTime=1e-08
  C6_lowered_switch : Switch  Criteria=u2 ~= 0  Threshold=double(0)  OutDataTypeStr=boolean  SampleTime=1e-08  SaturateOnIntegerOverflow=off  InputSameDT=off
  C7_lowered : Delay  DelayLength=double(1)  InitialCondition=0  SampleTime=1e-08
  C8_lowered : Delay  DelayLength=double(1)  InitialCondition=0  SampleTime=1e-08
  C8_lowered_Initial_Val : Constant  Value=double(1)  OutDataTypeStr=boolean  SampleTime=1e-08
  C8_lowered_ctrl_const : Constant  OutDataTypeStr=boolean  SampleTime=1e-08
  C8_lowered_ctrl_delay : Delay  DelayLength=double(1)  InitialCondition=0  SampleTime=1e-08
  C8_lowered_switch : Switch  Criteria=u2 ~= 0  Threshold=double(0)  OutDataTypeStr=boolean  SampleTime=1e-08  SaturateOnIntegerOverflow=off  InputSameDT=off
  C9_lowered : Delay  DelayLength=double(1)  InitialCondition=0  SampleTime=1e-08
  Delay{1,3..5} (4 alike) : Delay  DelayLength=double(1)  InitialCondition=0  SampleTime=1e-08
  From{1..46} (46 alike) : hdlmdlgenlib/Buffer
  Goto2 : hdlmdlgenlib/Buffer
  Goto3 : hdlmdlgenlib/Buffer
  Initial_Val{,2,4,6,8,10,13,15..16,18,20,22} (12 alike) : Constant  Value=double(0)  OutDataTypeStr=boolean  SampleTime=1e-08
  Initial_Val{1,3,5,7,9,11..12,14,17,19,21} (11 alike) : Constant  Value=double(1)  OutDataTypeStr=boolean  SampleTime=1e-08
  Logical Operator : Logic  Operator=XOR  AllPortsSameDT=off  OutDataTypeStr=boolean  SampleTime=1e-08
  Logical Operator1 : Logic  Operator=XOR  AllPortsSameDT=off  OutDataTypeStr=boolean  SampleTime=1e-08
  Sample Control Bus Creator : whdlutilities/Sample Control Bus Creator
  StateControl : StateControl  StateControl=Synchronous
  bus_selector : BusSelector  OutputSignals=start,end,valid
  enb_in{,1..22} (23 alike) : Switch  Criteria=u2 ~= 0  Threshold=double(0)  OutDataTypeStr=boolean  SampleTime=1e-08  SaturateOnIntegerOverflow=off  InputSameDT=off
  reset_in{,1..22} (23 alike) : Switch  Criteria=u2 ~= 0  Threshold=double(0)  OutDataTypeStr=boolean  SampleTime=1e-08  SaturateOnIntegerOverflow=off  InputSameDT=off
  data_out : Outport  SampleTime=1e-08
  ctrl_out : Outport  Port=2  SampleTime=1e-08
  wires:
  data_in/1 -> Delay1/1
  ctrl_in/1 -> bus_selector/1
  bus_selector/1 -> Goto3/1, Delay3/1  "<start>"
  bus_selector/2 -> Delay4/1  "<end>"
  bus_selector/3 -> Goto2/1, Delay5/1  "<valid>"
  Delay1/1 -> Logical Operator/1
  Delay3/1 -> Sample Control Bus Creator/1
  Delay4/1 -> Sample Control Bus Creator/2
  Delay5/1 -> Sample Control Bus Creator/3
  Logical Operator/1 -> data_out/1
  Logical Operator1/1 -> Logical Operator/2, enb_in/1
  Sample Control Bus Creator/1 -> ctrl_out/1
  Goto2/1 -> From8/1, From7/1, From5/1, From44/1, From42/1, From40/1, From38/1, From36/1, From34/1, From32/1, From30/1, From3/1, From28/1, From26/1, From24/1, From22/1, From20/1, From18/1, From16/1, From14/1, From12/1, From10/1, From1/1
  Goto3/1 -> From9/1, From6/1, From46/1, From45/1, From43/1, From41/1, From4/1, From39/1, From37/1, From35/1, From33/1, From31/1, From29/1, From27/1, From25/1, From23/1, From21/1, From2/1, From19/1, From17/1, From15/1, From13/1, From11/1
  C10_lowered_ctrl_const/1 -> C10_lowered_ctrl_delay/1
  C12_lowered_ctrl_const/1 -> C12_lowered_ctrl_delay/1
  C14_lowered_ctrl_const/1 -> C14_lowered_ctrl_delay/1
  C16_lowered_ctrl_const/1 -> C16_lowered_ctrl_delay/1
  C18_lowered_ctrl_const/1 -> C18_lowered_ctrl_delay/1
  C2_lowered_ctrl_const/1 -> C2_lowered_ctrl_delay/1
  C20_lowered_ctrl_const/1 -> C20_lowered_ctrl_delay/1
  C22_lowered_ctrl_const/1 -> C22_lowered_ctrl_delay/1
  C4_lowered_ctrl_const/1 -> C4_lowered_ctrl_delay/1
  C6_lowered_ctrl_const/1 -> C6_lowered_ctrl_delay/1
  C8_lowered_ctrl_const/1 -> C8_lowered_ctrl_delay/1
  C1_lowered/1 -> enb_in3/1, enb_in/3
  C19_lowered/1 -> enb_in5/1, enb_in2/3
  C3_lowered/1 -> enb_in7/1, enb_in4/3
  C21_lowered/1 -> enb_in9/1, enb_in6/3
  C5_lowered/1 -> enb_in11/1, enb_in8/3
  C23_lowered/1 -> enb_in10/3, Logical Operator1/1
  C7_lowered/1 -> enb_in13/1, enb_in12/3
  C9_lowered/1 -> enb_in15/1, enb_in14/3
  C11_lowered/1 -> enb_in17/1, enb_in16/3
  C13_lowered/1 -> enb_in19/1, enb_in18/3
  C15_lowered/1 -> enb_in21/1, enb_in20/3
  C17_lowered/1 -> enb_in22/3, enb_in1/1
  C18_lowered/1 -> C18_lowered_switch/1
  From7/1 -> enb_in/2
  Initial_Val/1 -> reset_in/1
  From46/1 -> reset_in/2
  From40/1 -> enb_in1/2
  Initial_Val9/1 -> reset_in1/1
  From41/1 -> reset_in1/2
  C18_lowered_ctrl_delay/1 -> C18_lowered_switch/2
  C18_lowered_Initial_Val/1 -> C18_lowered_switch/3
  From42/1 -> enb_in2/2
  Initial_Val10/1 -> reset_in2/1
  From43/1 -> reset_in2/2
  C2_lowered/1 -> C2_lowered_switch/1
  From1/1 -> enb_in3/2
  Initial_Val11/1 -> reset_in3/1
  From2/1 -> reset_in3/2
  C2_lowered_ctrl_delay/1 -> C2_lowered_switch/2
  C2_lowered_Initial_Val/1 -> C2_lowered_switch/3
  From3/1 -> enb_in4/2
  Initial_Val16/1 -> reset_in4/1
  From4/1 -> reset_in4/2
  C20_lowered/1 -> C20_lowered_switch/1
  From44/1 -> enb_in5/2
  Initial_Val12/1 -> reset_in5/1
  From45/1 -> reset_in5/2
  C20_lowered_ctrl_delay/1 -> C20_lowered_switch/2
  C20_lowered_Initial_Val/1 -> C20_lowered_switch/3
  From32/1 -> enb_in6/2
  Initial_Val13/1 -> reset_in6/1
  From33/1 -> reset_in6/2
  C4_lowered/1 -> C4_lowered_switch/1
  From5/1 -> enb_in7/2
  Initial_Val17/1 -> reset_in7/1
  From6/1 -> reset_in7/2
  C4_lowered_ctrl_delay/1 -> C4_lowered_switch/2
  C4_lowered_Initial_Val/1 -> C4_lowered_switch/3
  From8/1 -> enb_in8/2
  Initial_Val18/1 -> reset_in8/1
  From9/1 -> reset_in8/2
  C22_lowered/1 -> C22_lowered_switch/1
  From34/1 -> enb_in9/2
  Initial_Val14/1 -> reset_in9/1
  From35/1 -> reset_in9/2
  C22_lowered_ctrl_delay/1 -> C22_lowered_switch/2
  C22_lowered_Initial_Val/1 -> C22_lowered_switch/3
  From36/1 -> enb_in10/2
  Initial_Val15/1 -> reset_in10/1
  From37/1 -> reset_in10/2
  C6_lowered/1 -> C6_lowered_switch/1
  From10/1 -> enb_in11/2
  Initial_Val19/1 -> reset_in11/1
  From11/1 -> reset_in11/2
  C6_lowered_ctrl_delay/1 -> C6_lowered_switch/2
  C6_lowered_Initial_Val/1 -> C6_lowered_switch/3
  From12/1 -> enb_in12/2
  Initial_Val20/1 -> reset_in12/1
  From13/1 -> reset_in12/2
  C8_lowered/1 -> C8_lowered_switch/1
  From14/1 -> enb_in13/2
  Initial_Val21/1 -> reset_in13/1
  From15/1 -> reset_in13/2
  C8_lowered_ctrl_delay/1 -> C8_lowered_switch/2
  C8_lowered_Initial_Val/1 -> C8_lowered_switch/3
  From16/1 -> enb_in14/2
  Initial_Val22/1 -> reset_in14/1
  From17/1 -> reset_in14/2
  C10_lowered/1 -> C10_lowered_switch/1
  From24/1 -> enb_in15/2
  Initial_Val1/1 -> reset_in15/1
  From25/1 -> reset_in15/2
  C10_lowered_ctrl_delay/1 -> C10_lowered_switch/2
  C10_lowered_Initial_Val/1 -> C10_lowered_switch/3
  From26/1 -> enb_in16/2
  Initial_Val2/1 -> reset_in16/1
  From27/1 -> reset_in16/2
  C12_lowered/1 -> C12_lowered_switch/1
  From28/1 -> enb_in17/2
  Initial_Val3/1 -> reset_in17/1
  From29/1 -> reset_in17/2
  C12_lowered_ctrl_delay/1 -> C12_lowered_switch/2
  C12_lowered_Initial_Val/1 -> C12_lowered_switch/3
  From30/1 -> enb_in18/2
  Initial_Val4/1 -> reset_in18/1
  From31/1 -> reset_in18/2
  C14_lowered/1 -> C14_lowered_switch/1
  From18/1 -> enb_in19/2
  Initial_Val5/1 -> reset_in19/1
  From19/1 -> reset_in19/2
  C14_lowered_ctrl_delay/1 -> C14_lowered_switch/2
  C14_lowered_Initial_Val/1 -> C14_lowered_switch/3
  From20/1 -> enb_in20/2
  Initial_Val6/1 -> reset_in20/1
  From21/1 -> reset_in20/2
  C16_lowered/1 -> C16_lowered_switch/1
  From22/1 -> enb_in21/2
  Initial_Val7/1 -> reset_in21/1
  From23/1 -> reset_in21/2
  C16_lowered_ctrl_delay/1 -> C16_lowered_switch/2
  C16_lowered_Initial_Val/1 -> C16_lowered_switch/3
  From38/1 -> enb_in22/2
  Initial_Val8/1 -> reset_in22/1
  From39/1 -> reset_in22/2
  reset_in/1 -> C1_lowered/1
  reset_in1/1 -> C18_lowered/1
  reset_in2/1 -> C19_lowered/1
  enb_in/1 -> reset_in/3
  enb_in1/1 -> reset_in1/3
  C18_lowered_switch/1 -> Logical Operator1/2, enb_in2/1, enb_in1/3
  enb_in2/1 -> reset_in2/3
  reset_in5/1 -> C20_lowered/1
  reset_in6/1 -> C21_lowered/1
  enb_in5/1 -> reset_in5/3
  C20_lowered_switch/1 -> enb_in6/1, enb_in5/3
  enb_in6/1 -> reset_in6/3
  reset_in9/1 -> C22_lowered/1
  reset_in10/1 -> C23_lowered/1
  enb_in9/1 -> reset_in9/3
  C22_lowered_switch/1 -> enb_in10/1, enb_in9/3
  enb_in10/1 -> reset_in10/3
  reset_in3/1 -> C2_lowered/1
  reset_in4/1 -> C3_lowered/1
  enb_in3/1 -> reset_in3/3
  C2_lowered_switch/1 -> enb_in4/1, enb_in3/3
  enb_in4/1 -> reset_in4/3
  reset_in7/1 -> C4_lowered/1
  reset_in8/1 -> C5_lowered/1
  enb_in7/1 -> reset_in7/3
  C4_lowered_switch/1 -> enb_in8/1, enb_in7/3
  enb_in8/1 -> reset_in8/3
  reset_in11/1 -> C6_lowered/1
  reset_in12/1 -> C7_lowered/1
  enb_in11/1 -> reset_in11/3
  C6_lowered_switch/1 -> enb_in12/1, enb_in11/3
  enb_in12/1 -> reset_in12/3
  reset_in13/1 -> C8_lowered/1
  reset_in14/1 -> C9_lowered/1
  enb_in13/1 -> reset_in13/3
  C8_lowered_switch/1 -> enb_in14/1, enb_in13/3
  enb_in14/1 -> reset_in14/3
  reset_in15/1 -> C10_lowered/1
  reset_in16/1 -> C11_lowered/1
  enb_in15/1 -> reset_in15/3
  C10_lowered_switch/1 -> enb_in16/1, enb_in15/3
  enb_in16/1 -> reset_in16/3
  reset_in17/1 -> C12_lowered/1
  reset_in18/1 -> C13_lowered/1
  enb_in17/1 -> reset_in17/3
  C12_lowered_switch/1 -> enb_in18/1, enb_in17/3
  enb_in18/1 -> reset_in18/3
  reset_in19/1 -> C14_lowered/1
  reset_in20/1 -> C15_lowered/1
  enb_in19/1 -> reset_in19/3
  C14_lowered_switch/1 -> enb_in20/1, enb_in19/3
  enb_in20/1 -> reset_in20/3
  reset_in21/1 -> C16_lowered/1
  reset_in22/1 -> C17_lowered/1
  enb_in21/1 -> reset_in21/3
  C16_lowered_switch/1 -> enb_in22/1, enb_in21/3
  enb_in22/1 -> reset_in22/3

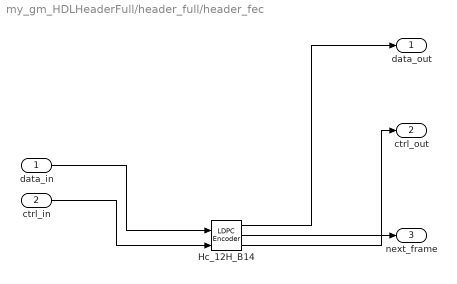
== system my_gm_HDLHeaderFull/header_full/header_fec ==
  data_in : Inport  OutDataTypeStr=boolean  SampleTime=1e-08
  ctrl_in : Inport  Port=2  SampleTime=1e-08
  Hc_12H_B14 : whdledac/LDPC Encoder  ParityCheckMatrix=Hc_12H  BlockSize=14  SimulateUsing=Code generation
  data_out : Outport  SampleTime=1e-08
  ctrl_out : Outport  Port=2  SampleTime=1e-08
  next_frame : Outport  Port=3  SampleTime=1e-08
  wires:
  data_in/1 -> Hc_12H_B14/1
  ctrl_in/1 -> Hc_12H_B14/2
  Hc_12H_B14/1 -> data_out/1
  Hc_12H_B14/2 -> ctrl_out/1
  Hc_12H_B14/3 -> next_frame/1

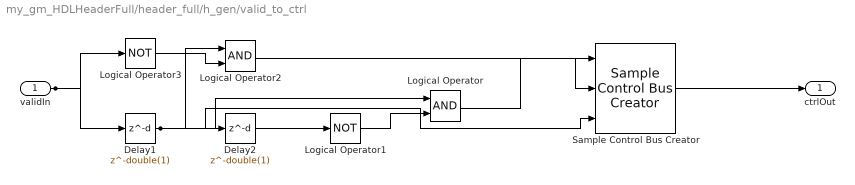
== system my_gm_HDLHeaderFull/header_full/h_gen/valid_to_ctrl ==
  validIn : Inport  OutDataTypeStr=boolean  SampleTime=1e-08
  Delay1 : Delay  DelayLength=double(1)  InitialCondition=0  SampleTime=1e-08
  Delay2 : Delay  DelayLength=double(1)  InitialCondition=0  SampleTime=1e-08
  Logical Operator : Logic  AllPortsSameDT=off  OutDataTypeStr=boolean  SampleTime=1e-08
  Logical Operator1 : Logic  Operator=NOT  Inputs=1  AllPortsSameDT=off  OutDataTypeStr=boolean  SampleTime=1e-08
  Logical Operator2 : Logic  AllPortsSameDT=off  OutDataTypeStr=boolean  SampleTime=1e-08
  Logical Operator3 : Logic  Operator=NOT  Inputs=1  AllPortsSameDT=off  OutDataTypeStr=boolean  SampleTime=1e-08
  Sample Control Bus Creator : whdlutilities/Sample Control Bus Creator
  ctrlOut : Outport  SampleTime=1e-08
  wires:
  validIn/1 -> Logical Operator3/1, Delay1/1
  Delay1/1 -> Logical Operator2/1, Logical Operator/1, Delay2/1, Sample Control Bus Creator/3
  Delay2/1 -> Logical Operator1/1
  Logical Operator/1 -> Sample Control Bus Creator/1
  Logical Operator1/1 -> Logical Operator/2
  Logical Operator2/1 -> Sample Control Bus Creator/2
  Logical Operator3/1 -> Logical Operator2/2
  Sample Control Bus Creator/1 -> ctrlOut/1
